simulink model "untitled"  (R2017b)
settings: Solver=VariableStepAuto  StartTime=0.0  StopTime=150  RelTol=1e-3
settings Model: Creator=zhonglinhong  LastModifiedBy=zhonglinhong

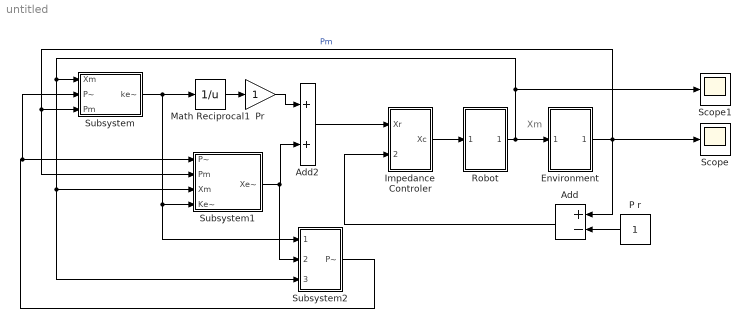
== system untitled ==
  note: Xm
  Add : Sum  Inputs=+-
  Add2 : Sum
  Environment : Subsystem  Tag=输入机器人末端位置x，输出由此产生的环境力。环境位置设置为x=1
  Impedance Controler : Subsystem  Tag=输入e和Xr
  Math Reciprocal1 : Math  Operator=reciprocal  SaturateOnIntegerOverflow=on
  P r : Constant
  Pr : Gain
  Robot : Subsystem  Tag=机器人末端执行器，输入控制位置Xc，输出测量位置Xm
  Scope : Scope
  Scope1 : Scope
  Subsystem : Subsystem
  Subsystem1 : Subsystem
  Subsystem2 : Subsystem
  wires:
  Robot/1(Out1) -> Subsystem/1(Xm), Subsystem2/3(Xm), Subsystem1/3(Xm), Scope1/1, Environment/1(In1)
  Environment/1(Out1) -> Subsystem/3(Pm), Subsystem1/2(Pm), Add/1, Scope/1  "Pm"
  P r/1 -> Add/2
  Add/1 -> Impedance Controler/2(error)
  Impedance Controler/1(Xc) -> Robot/1(In1)
  Subsystem/1(ke~) -> Subsystem2/1(Ke~), Subsystem1/4(Ke~), Math Reciprocal1/1
  Math Reciprocal1/1 -> Pr/1
  Pr/1 -> Add2/1
  Add2/1 -> Impedance Controler/1("Xr ")
  Subsystem1/1(Xe~) -> Subsystem2/2(Xe~), Add2/2
  Subsystem2/1(P~) -> Subsystem/2(P~), Subsystem1/1(P~)

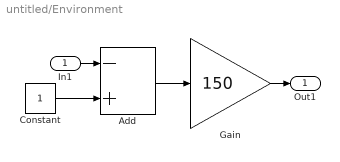
== system untitled/Environment ==
  In1 : Inport
  Add : Sum  Inputs=-+
  Constant : Constant
  Gain : Gain  Gain=150
  Out1 : Outport
  wires:
  Add/1 -> Gain/1
  In1/1 -> Add/1
  Gain/1 -> Out1/1
  Constant/1 -> Add/2

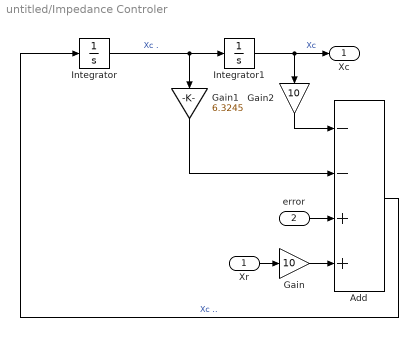
== system untitled/Impedance Controler ==
  "Xr " : Inport
  error : Inport  Port=2
  Add : Sum  Inputs=--++
  Gain : Gain  Gain=10
  Gain1 : Gain  Gain=6.3245
  Gain2 : Gain  Gain=10
  Integrator : Integrator
  Integrator1 : Integrator
  Xc : Outport
  wires:
  "Xr "/1 -> Gain/1
  Add/1 -> Integrator/1  "Xc .."
  Integrator/1 -> Gain1/1, Integrator1/1  "Xc ."
  error/1 -> Add/3
  Gain/1 -> Add/4
  Gain1/1 -> Add/2
  Integrator1/1 -> Xc/1, Gain2/1  "Xc"
  Gain2/1 -> Add/1

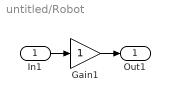
== system untitled/Robot ==
  In1 : Inport
  Gain1 : Gain
  Out1 : Outport
  wires:
  In1/1 -> Gain1/1
  Gain1/1 -> Out1/1

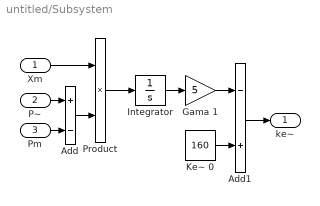
== system untitled/Subsystem ==
  Xm : Inport
  P~ : Inport  Port=2
  Pm : Inport  Port=3
  Add : Sum  Inputs=+-
  Add1 : Sum  Inputs=-+
  Gama 1 : Gain  Gain=5
  Integrator : Integrator
  "Ke~ 0 " : Constant  Value=160
  Product : Product
  ke~ : Outport
  wires:
  P~/1 -> Add/1
  Pm/1 -> Add/2
  Add/1 -> Product/2
  Xm/1 -> Product/1
  Product/1 -> Integrator/1
  Integrator/1 -> Gama 1/1
  Gama 1/1 -> Add1/1
  "Ke~ 0 "/1 -> Add1/2
  Add1/1 -> ke~/1

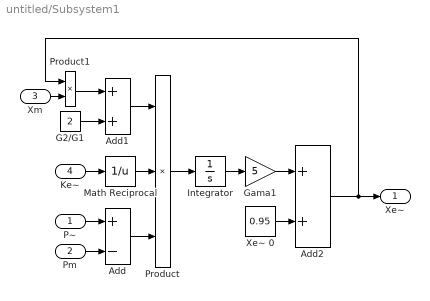
== system untitled/Subsystem1 ==
  P~ : Inport
  Pm : Inport  Port=2
  Xm : Inport  Port=3
  Ke~ : Inport  Port=4
  Add : Sum  Inputs=+-
  Add1 : Sum
  Add2 : Sum
  G2/G1 : Constant  Value=2
  Gama1 : Gain  Gain=5
  Integrator : Integrator
  Math Reciprocal : Math  Operator=reciprocal  SaturateOnIntegerOverflow=on
  Product : Product  Inputs=3
  Product1 : Product
  "Xe~ 0 " : Constant  Value=0.95
  Xe~ : Outport
  wires:
  Pm/1 -> Add/2
  P~/1 -> Add/1
  Ke~/1 -> Math Reciprocal/1
  Add/1 -> Product/3
  Math Reciprocal/1 -> Product/2
  Product/1 -> Integrator/1
  Integrator/1 -> Gama1/1
  "Xe~ 0 "/1 -> Add2/2
  Gama1/1 -> Add2/1
  Add2/1 -> Product1/1, Xe~/1
  Add1/1 -> Product/1
  Xm/1 -> Product1/2
  Product1/1 -> Add1/1
  G2/G1/1 -> Add1/2

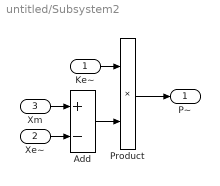
== system untitled/Subsystem2 ==
  Ke~ : Inport
  Xe~ : Inport  Port=2
  Xm : Inport  Port=3
  Add : Sum  Inputs=+-
  Product : Product
  P~ : Outport
  wires:
  Xe~/1 -> Add/2
  Xm/1 -> Add/1
  Add/1 -> Product/2
  Ke~/1 -> Product/1
  Product/1 -> P~/1
